simulink model "SAD_project"  (R2023b)
settings: Solver=ode4  StartTime=t0  StopTime=tf  FixedStep=t_step  RelTol=1e-3
model workspace (MAT data in the model file):
  N_order = 1
values from neighbouring files (symbols this model uses):
  A1 = importdata("igrfSg.txt")    [SAD_project_code.m]
  A2 = importdata("igrfSh.txt")    [SAD_project_code.m]
  A_1 = area_face(1)    [SAD_project_code.m]
  A_2 = area_face(2)    [SAD_project_code.m]
  A_3 = area_face(3)    [SAD_project_code.m]
  A_4 = area_face(4)    [SAD_project_code.m]
  A_5 = area_face(5)    [SAD_project_code.m]
  A_6 = area_face(6)    [SAD_project_code.m]
  alpha = [1/6 5/6]    [SAD_project_code.m]
  ARW = ARW*[1 1 1]'    [SAD_project_code.m]
  bias = bias*[1 1 1]'    [SAD_project_code.m]
  DCM_eci_per = rotationMatrix(rad2deg(i),rad2deg(OM), rad2deg(om))    [SAD_project_code.m]
  e = 0.0011241    [SAD_project_code.m]
  FS = 50000e-9    (= 5e-05)    [SAD_project_code.m]
  H0 = [g_10 g_11 h_11]'    [SAD_project_code.m]
  h_r_0 = [0,0,0]'    [SAD_project_code.m]
  horizon_cone_limit = deg2rad(350)    [SAD_project_code.m]
  i = deg2rad(97.55)    [SAD_project_code.m]
  I = 5/12.*diag([Ix Iy Iz])    [SAD_project_code.m]
  I_inv = inv(I)    [SAD_project_code.m]
  I_RW = 1e-2    (= 0.01)    [SAD_project_code.m]
  I_vector_RW = [I_RW I_RW I_RW]'    [SAD_project_code.m]
  inc_tot = sqrt(inc_lin^2 + inc_acc^2)    [SAD_project_code.m]
  InitialTrueAnomalyOfEarth = 0    [SAD_project_code.m]
  j_b = [0.001 0.005 0.001]'    [SAD_project_code.m]
  matrix_RW_config = eye(3)    [SAD_project_code.m]
  matrix_RW_config_inv = inv(matrix_RW_config)    [SAD_project_code.m]
  mu_E = astroConstants(13)    [SAD_project_code.m]
  N_1 = BODY(1,:)    [SAD_project_code.m]
  N_2 = BODY(2,:)    [SAD_project_code.m]
  N_3 = BODY(3,:)    [SAD_project_code.m]
  N_4 = BODY(4,:)    [SAD_project_code.m]
  N_5 = BODY(5,:)    [SAD_project_code.m]
  N_6 = BODY(6,:)    [SAD_project_code.m]
  n_e = sqrt(mu_E/a^3)    [SAD_project_code.m]
  om = deg2rad(206.3209)    [SAD_project_code.m]
  OM = deg2rad(50.7464)    [SAD_project_code.m]
  p = a*(1-e^2)    [SAD_project_code.m]
  q0 = [0.1, -0.7, 0.51, 0.41]    [SAD_project_code.m]
  r_1 = r(1,:)    [SAD_project_code.m]
  r_2 = r(2,:)    [SAD_project_code.m]
  r_3 = r(3,:)    [SAD_project_code.m]
  r_4 = r(4,:)    [SAD_project_code.m]
  r_5 = r(5,:)    [SAD_project_code.m]
  r_6 = r(6,:)    [SAD_project_code.m]
  R_E = astroConstants(23)    [SAD_project_code.m]
  rho_d1 = 0.1    [SAD_project_code.m]
  rho_d2 = 0.1    [SAD_project_code.m]
  rho_d3 = 0.1    [SAD_project_code.m]
  rho_d4 = 0.1    [SAD_project_code.m]
  rho_d5 = 0.1    [SAD_project_code.m]
  rho_d6 = 0.1    [SAD_project_code.m]
  rho_s1 = rho_s(1)    [SAD_project_code.m]
  rho_s2 = rho_s(2)    [SAD_project_code.m]
  rho_s3 = rho_s(3)    [SAD_project_code.m]
  rho_s4 = rho_s(4)    [SAD_project_code.m]
  rho_s5 = rho_s(5)    [SAD_project_code.m]
  rho_s6 = rho_s(6)    [SAD_project_code.m]
  t_step = 0.01    [SAD_project_code.m]
  th0 = deg2rad(0)    [SAD_project_code.m]
  timeoflaunch = date2mjd2000(date0)    [SAD_project_code.m]
  ts_sensor = 5*t_step    (= 0.05)    [SAD_project_code.m]
  w0 = [wx0 wy0 wz0]'    [SAD_project_code.m]
  w0_RW = [0 0 0]    [SAD_project_code.m]
  w_E = deg2rad(15.04)/60/60    [SAD_project_code.m]
  wMax_RW = 2*pi * RPM_max_RW / 60    (= 527.263967027)    [SAD_project_code.m]
libraries: matrix_library x21, simulink x5, simulink_extras x4, dspindex x3, vrlib x2, aerolibutil x1
(part 2 of 3)

== system SAD_project/Statistical methods attitude determination (quaternion  Wabha’s problem) /Vector z ==
  B : Inport
  Gain1 : Gain  Gain=-1
  Selector : Selector  NumberOfDimensions=2  InputPortWidth=3  IndexOptions=Index vector (dialog),Starting index (dialog)  Indices=2,3  OutputSizes=1,1
  Selector1 : Selector  NumberOfDimensions=2  InputPortWidth=3  IndexOptions=Index vector (dialog),Starting index (dialog)  Indices=1,3  OutputSizes=1,1
  Selector2 : Selector  NumberOfDimensions=2  InputPortWidth=3  IndexOptions=Index vector (dialog),Starting index (dialog)  Indices=1,2  OutputSizes=1,1
  Subtract1 : Sum  Inputs=+-
  Transpose1 : Math  Operator=transpose
  Vector Concatenate : Concatenate  NumInputs=3
  z : Outport
  wires:
  B/1 -> Subtract1/1, Transpose1/1
  Transpose1/1 -> Subtract1/2
  Selector2/1 -> Vector Concatenate/3
  Selector/1 -> Vector Concatenate/1
  Subtract1/1 -> Selector/1, Selector2/1, Selector1/1
  Vector Concatenate/1 -> z/1
  Gain1/1 -> Vector Concatenate/2
  Selector1/1 -> Gain1/1

== system SAD_project/Subsystem/Switch Case Action Adavanced Magnetic model ==
  r_N : Inport
  Action Port : ActionPort  PropagateVarSize=During execution  ActionPortLabel=case [ 1 ]:
  Advanced magnetic field model : Subsystem
  Constant : Constant  Value=N_order
  Gain : Gain  Gain=10^(-9)
  B_n : Outport  VectorParamsAs1DForOutWhenUnconnected=off
  wires:
  r_N/1 -> Advanced magnetic field model/1(r_N)
  Advanced magnetic field model/1(B_n) -> Gain/1
  Gain/1 -> B_n/1
  Constant/1 -> Advanced magnetic field model/2(N order)

== system SAD_project/Subsystem/Switch Case Action Dipole model ==
  r_N : Inport
  Action Port : ActionPort  PropagateVarSize=During execution  ActionPortLabel=default:
  Dipol Model of Magnetic Field : Subsystem
  Gain : Gain  Gain=10^(-9)
  "[g0_1, g1_1, h1_1]" : Constant  Value=H0
  b_N : Outport  VectorParamsAs1DForOutWhenUnconnected=off
  wires:
  "[g0_1, g1_1, h1_1]"/1 -> Dipol Model of Magnetic Field/1(H0 vector)
  r_N/1 -> Dipol Model of Magnetic Field/2(EarthSat_n)
  Dipol Model of Magnetic Field/1(b_N) -> Gain/1
  Gain/1 -> b_N/1

== system SAD_project/Sun sensor (Da fare sistmando vettore e eclissi)/Normalize Vector1 ==
  Vector : Inport
  Divide : Product  Inputs=*/
  Normalize Vector : Subsystem  AncestorBlock=LibrarySAD5/Normalize Vector1
  Versor : Outport
  wires:
  Vector/1 -> Normalize Vector/1(Vector), Divide/1
  Divide/1 -> Versor/1
  Normalize Vector/1(Norm) -> Divide/2

== system SAD_project/TRIAD: Attitude determination algebric Method with 2 sensor/Normalize Vector1 ==
  Vector : Inport
  Divide : Product  Inputs=*/
  Normalize Vector : Subsystem  AncestorBlock=LibrarySAD5/Normalize Vector1
  Versor : Outport
  wires:
  Vector/1 -> Normalize Vector/1(Vector), Divide/1
  Divide/1 -> Versor/1
  Normalize Vector/1(Norm) -> Divide/2

== system SAD_project/TRIAD: Attitude determination algebric Method with 2 sensor/Normalize Vector2 ==
  Vector : Inport
  Divide : Product  Inputs=*/
  Normalize Vector : Subsystem  AncestorBlock=LibrarySAD5/Normalize Vector1
  Versor : Outport
  wires:
  Vector/1 -> Normalize Vector/1(Vector), Divide/1
  Divide/1 -> Versor/1
  Normalize Vector/1(Norm) -> Divide/2

== system SAD_project/TRIAD: Attitude determination algebric Method with 2 sensor/Normalize Vector3 ==
  Vector : Inport
  Divide : Product  Inputs=*/
  Normalize Vector : Subsystem  AncestorBlock=LibrarySAD5/Normalize Vector1
  Versor : Outport
  wires:
  Vector/1 -> Normalize Vector/1(Vector), Divide/1
  Divide/1 -> Versor/1
  Normalize Vector/1(Norm) -> Divide/2

== system SAD_project/TRIAD: Attitude determination algebric Method with 2 sensor/Normalize Vector4 ==
  Vector : Inport
  Divide : Product  Inputs=*/
  Normalize Vector : Subsystem  AncestorBlock=LibrarySAD5/Normalize Vector1
  Versor : Outport
  wires:
  Vector/1 -> Normalize Vector/1(Vector), Divide/1
  Divide/1 -> Versor/1
  Normalize Vector/1(Norm) -> Divide/2

== system SAD_project/TRIAD: Attitude determination algebric Method with 2 sensor/Subsystem ==
  note: S1 = 𝑝;
      | 𝑠2 = (𝑝 ∧ 𝑞)/(|𝑝 ∧ 𝑞|);
      | 𝑠3 = 𝑝 ∧ 𝑠2
  versor p (body frame) : Inport
  versor q (body frame) : Inport  Port=2
  Cross Product : matrix_library/Cross Product
  Cross Product1 : matrix_library/Cross Product
  Matrix Concatenate : Concatenate  NumInputs=3  Mode=Multidimensional array  ConcatenateDimension=2
  Normalize Vector3 : Subsystem
  "Matrix S Measurements " : Outport
  wires:
  versor q (body frame)/1 -> Cross Product/2
  Normalize Vector3/1(Versor) -> Matrix Concatenate/2, Cross Product1/2  "s2"
  versor p (body frame)/1 -> Cross Product1/1, Matrix Concatenate/1, Cross Product/1  "s1"
  Cross Product/1 -> Normalize Vector3/1(Vector)
  Cross Product1/1 -> Matrix Concatenate/3  "s3"
  Matrix Concatenate/1 -> "Matrix S Measurements "/1  "Matrix of measure in body frame"

== system SAD_project/TRIAD: Attitude determination algebric Method with 2 sensor/Subsystem1 ==
  versor a (body frame) : Inport
  versor b (body frame) : Inport  Port=2
  Cross Product : matrix_library/Cross Product
  Cross Product1 : matrix_library/Cross Product
  Matrix Concatenate : Concatenate  NumInputs=3  Mode=Multidimensional array  ConcatenateDimension=2
  Normalize Vector3 : Subsystem
  "Matrix V certain model " : Outport
  wires:
  versor b (body frame)/1 -> Cross Product/2
  Normalize Vector3/1(Versor) -> Matrix Concatenate/2, Cross Product1/2  "s2"
  versor a (body frame)/1 -> Cross Product1/1, Matrix Concatenate/1, Cross Product/1  "s1"
  Cross Product/1 -> Normalize Vector3/1(Vector)
  Cross Product1/1 -> Matrix Concatenate/3  "s3"
  Matrix Concatenate/1 -> "Matrix V certain model "/1  "Matrix of measure in body frame"

== system SAD_project/two-body Keplerian dynamics ECI/Integretion of true anomaly ==
  th0 : Inport
  (1-e^2)^(3/2) : Subsystem
  Constant : Constant
  Cos : Trigonometry  Operator=cos
  Divide : Product  Inputs=*/
  Gain : Gain  Gain=e
  Gain1 : Gain  Gain=n_e
  Integrator : Integrator  InitialConditionSource=external
  Product : Product
  Sum : Sum  Inputs=|++
  th : Outport
  wires:
  Sum/1 -> Product/1, Product/2
  Integrator/1 -> th/1, Cos/1  "theta"
  Divide/1 -> Integrator/1
  Constant/1 -> Sum/1
  Product/1 -> Gain1/1
  Cos/1 -> Gain/1
  Gain/1 -> Sum/2
  (1-e^2)^(3/2)/1(Out1) -> Divide/2
  th0/1 -> Integrator/2
  Gain1/1 -> Divide/1

== system SAD_project/two-body Keplerian dynamics ECI/r_perifocal ==
  th : Inport
  Calculation of norm r : Subsystem
  Constant : Constant  Value=0
  Cos : Trigonometry  Operator=cos
  Mux : Mux  Inputs=3
  Product : Product
  Sin : Trigonometry
  r_per : Outport
  wires:
  Constant/1 -> Mux/3
  Cos/1 -> Mux/1
  th/1 -> Calculation of norm r/1(th), Cos/1, Sin/1
  Sin/1 -> Mux/2
  Mux/1 -> Product/1  "r_n"
  Calculation of norm r/1(Norm(r)) -> Product/2
  Product/1 -> r_per/1  "r_n"

== system SAD_project/Calculation of disturbance torque/M of gravity gradient1/Norm of vector ==
  Vector : Inport
  Dot Product : DotProduct  OutDataTypeStr=Inherit: Inherit via internal rule
  Sqrt : Sqrt
  Norm : Outport
  wires:
  Sqrt/1 -> Norm/1
  Vector/1 -> Dot Product/1, Dot Product/2
  Dot Product/1 -> Sqrt/1

== system SAD_project/Calculation of disturbance torque/Solar pressure on 6 faces/Norm of vector ==
  Vector : Inport
  Dot Product : DotProduct  OutDataTypeStr=Inherit: Inherit via internal rule
  Sqrt : Sqrt
  Norm : Outport
  wires:
  Sqrt/1 -> Norm/1
  Vector/1 -> Dot Product/1, Dot Product/2
  Dot Product/1 -> Sqrt/1

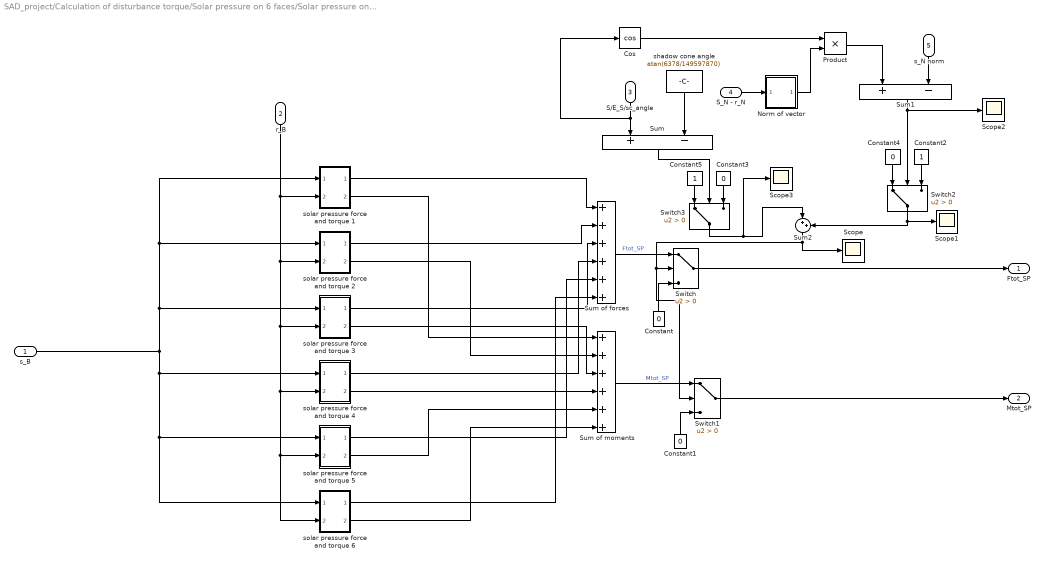
== system SAD_project/Calculation of disturbance torque/Solar pressure on 6 faces/Solar pressure on 6 faces1 ==
  s_B : Inport
  r_B : Inport  Port=2
  S/E_S/sc_angle : Inport  Port=3
  S_N - r_N : Inport  Port=4
  s_N norm : Inport  Port=5
  Constant{,1,3..4} (4 alike) : Constant  Value=0
  Constant2 : Constant
  Constant5 : Constant
  Cos : Trigonometry  Operator=cos
  Norm of vector : Subsystem  AncestorBlock=LibrarySAD5/Normalize Vector1
  Product : Product
  Scope{,1..3} (4 alike) : Scope
  Sum : Sum  Inputs=+-
  Sum of forces : Sum  Inputs=++++++
  Sum of moments : Sum  Inputs=++++++
  Sum1 : Sum  Inputs=+-
  Sum2 : Sum  Inputs=|++
  Switch{,1..3} (4 alike) : Switch  Criteria=u2 > Threshold  SaturateOnIntegerOverflow=off  InputSameDT=off
  shadow cone angle : Constant  Value=atan(6378/149597870)
  solar pressure force and torque 1 : Subsystem
  solar pressure force and torque 2 : Subsystem
  solar pressure force and torque 3 : Subsystem
  solar pressure force and torque 4 : Subsystem
  solar pressure force and torque 5 : Subsystem
  solar pressure force and torque 6 : Subsystem
  Ftot_SP : Outport
  Mtot_SP : Outport  Port=2
  wires:
  s_B/1 -> solar pressure force and torque 1/1(s_B), solar pressure force and torque 2/1(s_B), solar pressure force and torque 3/1(s_B), solar pressure force and torque 4/1(s_B), solar pressure force and torque 6/1(s_B), solar pressure force and torque 5/1(s_B)
  solar pressure force and torque 1/1(F_1) -> Sum of forces/1
  solar pressure force and torque 1/2(M_1) -> Sum of moments/1
  solar pressure force and torque 2/1(F_2) -> Sum of forces/2
  r_B/1 -> solar pressure force and torque 6/2(r_N), solar pressure force and torque 5/2(r_N), solar pressure force and torque 4/2(r_N), solar pressure force and torque 3/2(r_N), solar pressure force and torque 2/2(r_N), solar pressure force and torque 1/2(r_N)
  solar pressure force and torque 2/2(M_2) -> Sum of moments/2
  solar pressure force and torque 3/1(F_3) -> Sum of forces/3
  solar pressure force and torque 3/2(M_3) -> Sum of moments/3
  solar pressure force and torque 4/1(F_4) -> Sum of forces/4
  solar pressure force and torque 4/2(M_4) -> Sum of moments/4
  solar pressure force and torque 5/1(F_5) -> Sum of forces/5
  solar pressure force and torque 5/2(M_5) -> Sum of moments/5
  solar pressure force and torque 6/1(F_6) -> Sum of forces/6
  solar pressure force and torque 6/2(M_6) -> Sum of moments/6
  Sum of forces/1 -> Switch/1  "Ftot_SP"
  Constant/1 -> Switch/3
  S/E_S/sc_angle/1 -> Cos/1, Sum/1
  shadow cone angle/1 -> Sum/2
  Sum of moments/1 -> Switch1/1  "Mtot_SP"
  Constant1/1 -> Switch1/3
  S_N - r_N/1 -> Norm of vector/1(Vector)
  Constant2/1 -> Switch2/3
  Cos/1 -> Product/1
  Norm of vector/1(Norm) -> Product/2
  Product/1 -> Sum1/1
  s_N norm/1 -> Sum1/2
  Sum/1 -> Switch3/2
  Sum1/1 -> Switch2/2, Scope2/1
  Constant4/1 -> Switch2/1
  Constant5/1 -> Switch3/1
  Constant3/1 -> Switch3/3
  Switch3/1 -> Scope3/1, Sum2/1
  Switch2/1 -> Sum2/2, Scope1/1
  Sum2/1 -> Scope/1, Switch1/2, Switch/2
  Switch/1 -> Ftot_SP/1
  Switch1/1 -> Mtot_SP/1

== system SAD_project/Create matrix to statistical method/Normalize Vector1/Normalize Vector ==
  Vector : Inport
  Dot Product : DotProduct  OutDataTypeStr=Inherit: Inherit via internal rule
  Sqrt : Sqrt
  Norm : Outport
  wires:
  Sqrt/1 -> Norm/1
  Vector/1 -> Dot Product/1, Dot Product/2
  Dot Product/1 -> Sqrt/1

== system SAD_project/Create matrix to statistical method/Normalize Vector2/Normalize Vector ==
  Vector : Inport
  Dot Product : DotProduct  OutDataTypeStr=Inherit: Inherit via internal rule
  Sqrt : Sqrt
  Norm : Outport
  wires:
  Sqrt/1 -> Norm/1
  Vector/1 -> Dot Product/1, Dot Product/2
  Dot Product/1 -> Sqrt/1

== system SAD_project/Create matrix to statistical method/Normalize Vector3/Normalize Vector ==
  Vector : Inport
  Dot Product : DotProduct  OutDataTypeStr=Inherit: Inherit via internal rule
  Sqrt : Sqrt
  Norm : Outport
  wires:
  Sqrt/1 -> Norm/1
  Vector/1 -> Dot Product/1, Dot Product/2
  Dot Product/1 -> Sqrt/1

== system SAD_project/Create matrix to statistical method/Normalize Vector4/Normalize Vector ==
  Vector : Inport
  Dot Product : DotProduct  OutDataTypeStr=Inherit: Inherit via internal rule
  Sqrt : Sqrt
  Norm : Outport
  wires:
  Sqrt/1 -> Norm/1
  Vector/1 -> Dot Product/1, Dot Product/2
  Dot Product/1 -> Sqrt/1

== system SAD_project/Dynamics e Kinematics/Attitude error GG/calculating A_B//L ==
  Theta : Inport
  A_B/N : Inport  Port=2
  Matrix Multiply : Product  Multiplication=Matrix(*)
  Subsystem : Subsystem
  Transpose : Math  Operator=transpose
  A_B/L : Outport
  wires:
  Theta/1 -> Subsystem/1(Theta)
  Transpose/1 -> Matrix Multiply/2
  A_B/N/1 -> Matrix Multiply/1
  Matrix Multiply/1 -> A_B/L/1
  Subsystem/1(" A_L/N") -> Transpose/1

== system SAD_project/Dynamics e Kinematics/DCM composition from quaternions 1/Cross product matrix composition ==
  q_vect : Inport
  Demux : Demux  Outputs=3
  Gain : Gain  Gain=[0 0 0; 0 0 -1; 0 1 0]
  Gain1 : Gain  Gain=[0 0 1; 0 0 0; -1 0 0]
  Gain2 : Gain  Gain=[0 -1 0; 1 0 0; 0 0 0]
  Sum : Sum  Inputs=+++
  q_vect cross : Outport
  wires:
  Gain1/1 -> Sum/2
  Demux/3 -> Gain2/1
  Demux/1 -> Gain/1
  q_vect/1 -> Demux/1
  Gain2/1 -> Sum/3
  Demux/2 -> Gain1/1
  Gain/1 -> Sum/1
  Sum/1 -> q_vect cross/1

== system SAD_project/Dynamics e Kinematics/Kinematics quaternion2/Matrix OMEGA ==
  omega : Inport
  Constant4 : Constant  Value=0
  Demux : Demux  Outputs=3
  Gain : Gain  Gain=-1
  Gain1 : Gain  Gain=-1
  Gain2 : Gain  Gain=-1
  Matrix Concatenate : Concatenate  NumInputs=4  Mode=Multidimensional array  ConcatenateDimension=2
  Vector Concatenate{,2..4} (4 alike) : Concatenate  NumInputs=4
  Matrix Omega : Outport
  wires:
  Demux/2 -> Vector Concatenate4/2, Vector Concatenate/3, Gain1/1  "W_v"
  Gain1/1 -> Vector Concatenate2/4, Vector Concatenate3/1
  Matrix Concatenate/1 -> Matrix Omega/1
  Gain2/1 -> Vector Concatenate3/4, Vector Concatenate/2  "-W_w"
  Vector Concatenate3/1 -> Matrix Concatenate/3
  Demux/3 -> Vector Concatenate2/1, Vector Concatenate4/3, Gain2/1  "W_w"
  Gain/1 -> Vector Concatenate/4, Vector Concatenate2/3  "-W_u"
  Constant4/1 -> Vector Concatenate/1, Vector Concatenate2/2, Vector Concatenate3/3, Vector Concatenate4/4
  Demux/1 -> Vector Concatenate3/2, Vector Concatenate4/1, Gain/1  "W_u"
  Vector Concatenate4/1 -> Matrix Concatenate/4
  Vector Concatenate2/1 -> Matrix Concatenate/2
  Vector Concatenate/1 -> Matrix Concatenate/1
  omega/1 -> Demux/1

== system SAD_project/Dynamics e Kinematics/Kinematics quaternion2/Normalize Vector2 ==
  Vector : Inport
  Dot Product : DotProduct  OutDataTypeStr=Inherit: Inherit via internal rule
  Sqrt : Sqrt
  Norm : Outport
  wires:
  Sqrt/1 -> Norm/1
  Vector/1 -> Dot Product/1, Dot Product/2
  Dot Product/1 -> Sqrt/1

== system SAD_project/Horizon Sensor/Normalize Vector1/Normalize Vector ==
  Vector : Inport
  Dot Product : DotProduct  OutDataTypeStr=Inherit: Inherit via internal rule
  Sqrt : Sqrt
  Norm : Outport
  wires:
  Sqrt/1 -> Norm/1
  Vector/1 -> Dot Product/1, Dot Product/2
  Dot Product/1 -> Sqrt/1

== system SAD_project/Subsystem/Switch Case Action Adavanced Magnetic model/Advanced magnetic field model ==
  note: INPUT:
      | - r_N are the coordinates of the satellite in the ECI frame
      | - A_bn is the DCM matrix to change from inertial frame to body frame
      | - timeoflaunch is the julian time at the start of simulation
      | - A1 and A2 are the matrices containing the coefficients of g and h up to the 13th order
      | - j_B is the residual magnetic induction
  note: the timeoflaunch is corrected by adding the time of simulation using a clock
  r_N : Inport
  N order : Inport  Port=2
  Clock1 : Clock
  Constant21 : Constant  Value=timeoflaunch
  Constant23 : Constant  Value=A1
  Constant24 : Constant  Value=A2
  Gain1 : Gain  Gain=1/(3600*24)
  MATLAB Function : MATLAB Function  TreatAsAtomicUnit=on
  Product3 : Product  Multiplication=Matrix(*)
  Rotation matrix for earth spin : Subsystem
  Sum : Sum  Inputs=|++
  cart to sph coord : Subsystem
  B_n : Outport
  wires:
  Rotation matrix for earth spin/1(eci_to_ecef) -> Product3/1
  Clock1/1 -> Gain1/1
  r_N/1 -> Product3/2
  Constant24/1 -> MATLAB Function/7(A2)
  cart to sph coord/3(long) -> MATLAB Function/4(LST), MATLAB Function/3(phi)
  Constant23/1 -> MATLAB Function/6(A1)
  Gain1/1 -> Sum/2
  Product3/1 -> cart to sph coord/1(r_xyz)
  cart to sph coord/2(lat) -> MATLAB Function/2(theta)
  Constant21/1 -> Sum/1
  Sum/1 -> MATLAB Function/5(mjd2000)
  cart to sph coord/1(r) -> MATLAB Function/1(r)
  MATLAB Function/1(B_n) -> B_n/1
  N order/1 -> MATLAB Function/8(N)

== system SAD_project/Subsystem/Switch Case Action Dipole model/Dipol Model of Magnetic Field ==
  note: CODE TO ADD
      | % Definition of Magnetic Field (Dipole model)
      |  j_b = [0.01 0.05 0.01]';
      | H0 = 1e-9.*[-29404.8 -1450.9 4652.5]';
  H0 vector : Inport
  EarthSat_n : Inport  Port=2
  Calculation of b_n : Subsystem
  b_N : Outport
  wires:
  H0 vector/1 -> Calculation of b_n/1(H0 vector)
  EarthSat_n/1 -> Calculation of b_n/2(EarthSat_n)
  Calculation of b_n/1(b_N) -> b_N/1

== system SAD_project/Sun sensor (Da fare sistmando vettore e eclissi)/Normalize Vector1/Normalize Vector ==
  Vector : Inport
  Dot Product : DotProduct  OutDataTypeStr=Inherit: Inherit via internal rule
  Sqrt : Sqrt
  Norm : Outport
  wires:
  Sqrt/1 -> Norm/1
  Vector/1 -> Dot Product/1, Dot Product/2
  Dot Product/1 -> Sqrt/1

== system SAD_project/TRIAD: Attitude determination algebric Method with 2 sensor/Normalize Vector1/Normalize Vector ==
  Vector : Inport
  Dot Product : DotProduct  OutDataTypeStr=Inherit: Inherit via internal rule
  Sqrt : Sqrt
  Norm : Outport
  wires:
  Sqrt/1 -> Norm/1
  Vector/1 -> Dot Product/1, Dot Product/2
  Dot Product/1 -> Sqrt/1

== system SAD_project/TRIAD: Attitude determination algebric Method with 2 sensor/Normalize Vector2/Normalize Vector ==
  Vector : Inport
  Dot Product : DotProduct  OutDataTypeStr=Inherit: Inherit via internal rule
  Sqrt : Sqrt
  Norm : Outport
  wires:
  Sqrt/1 -> Norm/1
  Vector/1 -> Dot Product/1, Dot Product/2
  Dot Product/1 -> Sqrt/1

== system SAD_project/TRIAD: Attitude determination algebric Method with 2 sensor/Normalize Vector3/Normalize Vector ==
  Vector : Inport
  Dot Product : DotProduct  OutDataTypeStr=Inherit: Inherit via internal rule
  Sqrt : Sqrt
  Norm : Outport
  wires:
  Sqrt/1 -> Norm/1
  Vector/1 -> Dot Product/1, Dot Product/2
  Dot Product/1 -> Sqrt/1

== system SAD_project/TRIAD: Attitude determination algebric Method with 2 sensor/Normalize Vector4/Normalize Vector ==
  Vector : Inport
  Dot Product : DotProduct  OutDataTypeStr=Inherit: Inherit via internal rule
  Sqrt : Sqrt
  Norm : Outport
  wires:
  Sqrt/1 -> Norm/1
  Vector/1 -> Dot Product/1, Dot Product/2
  Dot Product/1 -> Sqrt/1

== system SAD_project/TRIAD: Attitude determination algebric Method with 2 sensor/Subsystem/Normalize Vector3 ==
  Vector : Inport
  Divide : Product  Inputs=*/
  Normalize Vector : Subsystem  AncestorBlock=LibrarySAD5/Normalize Vector1
  Versor : Outport
  wires:
  Vector/1 -> Normalize Vector/1(Vector), Divide/1
  Divide/1 -> Versor/1
  Normalize Vector/1(Norm) -> Divide/2

== system SAD_project/TRIAD: Attitude determination algebric Method with 2 sensor/Subsystem1/Normalize Vector3 ==
  Vector : Inport
  Divide : Product  Inputs=*/
  Normalize Vector : Subsystem  AncestorBlock=LibrarySAD5/Normalize Vector1
  Versor : Outport
  wires:
  Vector/1 -> Normalize Vector/1(Vector), Divide/1
  Divide/1 -> Versor/1
  Normalize Vector/1(Norm) -> Divide/2

== system SAD_project/two-body Keplerian dynamics ECI/Integretion of true anomaly/(1-e^2)^(3//2) ==
  Constant1 : Constant
  Constant2 : Constant  Value=e
  Constant3 : Constant  Value=3/2
  Power : Math  Operator=pow
  Product1 : Product
  Subtract : Sum  Inputs=+-
  Out1 : Outport
  wires:
  Constant3/1 -> Power/2
  Constant2/1 -> Product1/2, Product1/1
  Subtract/1 -> Power/1
  Constant1/1 -> Subtract/1
  Product1/1 -> Subtract/2
  Power/1 -> Out1/1

== system SAD_project/two-body Keplerian dynamics ECI/r_perifocal/Calculation of norm r ==
  th : Inport
  Constant : Constant  Value=p
  Constant2 : Constant
  Cos : Trigonometry  Operator=cos
  Divide : Product  Inputs=*/
  Gain1 : Gain  Gain=e
  Sum : Sum  Inputs=|++
  Norm(r) : Outport
  wires:
  Constant/1 -> Divide/1
  Gain1/1 -> Sum/2
  Constant2/1 -> Sum/1
  Cos/1 -> Gain1/1
  Sum/1 -> Divide/2
  th/1 -> Cos/1
  Divide/1 -> Norm(r)/1

== system SAD_project/Calculation of disturbance torque/Solar pressure on 6 faces/Solar pressure on 6 faces1/Norm of vector ==
  Vector : Inport
  Dot Product : DotProduct  OutDataTypeStr=Inherit: Inherit via internal rule
  Sqrt : Sqrt
  Norm : Outport
  wires:
  Sqrt/1 -> Norm/1
  Vector/1 -> Dot Product/1, Dot Product/2
  Dot Product/1 -> Sqrt/1

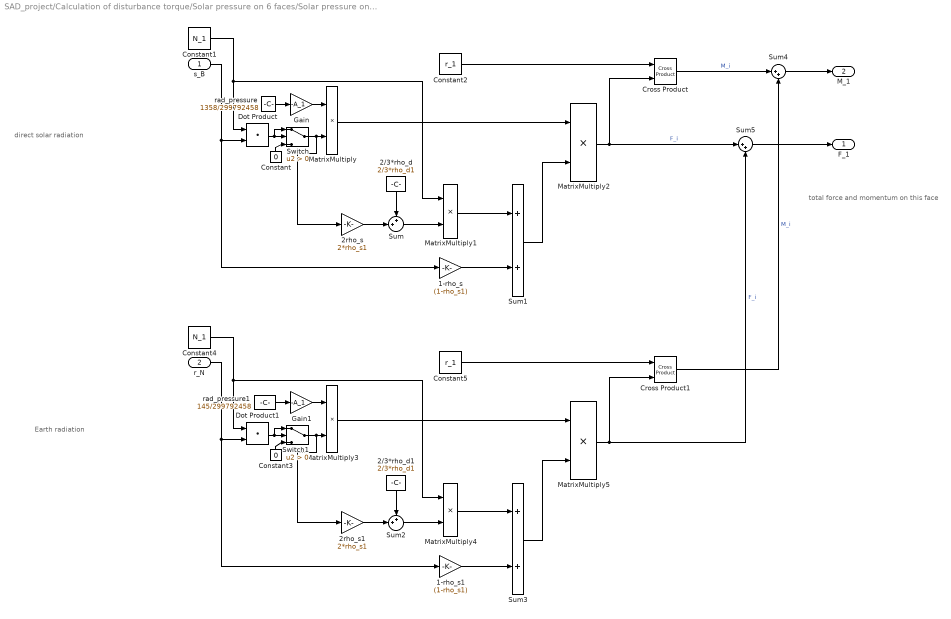
== system SAD_project/Calculation of disturbance torque/Solar pressure on 6 faces/Solar pressure on 6 faces1/solar pressure force and torque 1 ==
  note: total force and
      | momentum on this face
  note: direct solar radiation
  note: Earth radiation
  s_B : Inport
  r_N : Inport  Port=2
  1-rho_s : Gain  Gain=(1-rho_s1)
  1-rho_s1 : Gain  Gain=(1-rho_s1)
  2/3*rho_d : Constant  Value=2/3*rho_d1
  2/3*rho_d1 : Constant  Value=2/3*rho_d1
  2rho_s : Gain  Gain=2*rho_s1
  2rho_s1 : Gain  Gain=2*rho_s1
  Constant : Constant  Value=0
  Constant1 : Constant  Value=N_1
  Constant2 : Constant  Value=r_1
  Constant3 : Constant  Value=0
  Constant4 : Constant  Value=N_1
  Constant5 : Constant  Value=r_1
  Cross Product : matrix_library/Cross Product
  Cross Product1 : matrix_library/Cross Product
  Dot Product : DotProduct  OutDataTypeStr=Inherit: Inherit via internal rule
  Dot Product1 : DotProduct  OutDataTypeStr=Inherit: Inherit via internal rule
  Gain : Gain  Gain=-A_1
  Gain1 : Gain  Gain=-A_1
  MatrixMultiply{,1..5} (6 alike) : Product
  Sum : Sum  Inputs=++|
  Sum1 : Sum
  Sum2 : Sum  Inputs=++|
  Sum3 : Sum
  Sum4 : Sum  Inputs=|++
  Sum5 : Sum  Inputs=|++
  Switch : Switch  Criteria=u2 > Threshold  SaturateOnIntegerOverflow=off  InputSameDT=off
  Switch1 : Switch  Criteria=u2 > Threshold  SaturateOnIntegerOverflow=off  InputSameDT=off
  rad_pressure : Constant  Value=1358/299792458
  rad_pressure1 : Constant  Value=145/299792458
  F_1 : Outport
  M_1 : Outport  Port=2
  wires:
  MatrixMultiply2/1 -> Sum5/1, Cross Product/2  "F_i"
  MatrixMultiply/1 -> MatrixMultiply2/1
  Sum1/1 -> MatrixMultiply2/2
  s_B/1 -> 1-rho_s/1, Dot Product/2
  1-rho_s/1 -> Sum1/2
  rad_pressure/1 -> Gain/1
  MatrixMultiply1/1 -> Sum1/1
  Constant1/1 -> MatrixMultiply1/1, Dot Product/1
  Gain/1 -> MatrixMultiply/1
  Constant2/1 -> Cross Product/1
  Dot Product/1 -> Switch/1, Switch/2
  Constant/1 -> Switch/3
  Switch/1 -> 2rho_s/1, MatrixMultiply/2
  2rho_s/1 -> Sum/2
  2/3*rho_d/1 -> Sum/1
  Sum/1 -> MatrixMultiply1/2
  Sum3/1 -> MatrixMultiply5/2
  r_N/1 -> 1-rho_s1/1, Dot Product1/2
  1-rho_s1/1 -> Sum3/2
  2rho_s1/1 -> Sum2/2
  Switch1/1 -> 2rho_s1/1, MatrixMultiply3/2
  MatrixMultiply4/1 -> Sum3/1
  Constant5/1 -> Cross Product1/1
  MatrixMultiply3/1 -> MatrixMultiply5/1
  rad_pressure1/1 -> Gain1/1
  Constant3/1 -> Switch1/3
  Constant4/1 -> MatrixMultiply4/1, Dot Product1/1
  MatrixMultiply5/1 -> Sum5/2, Cross Product1/2  "F_i"
  Dot Product1/1 -> Switch1/1, Switch1/2
  Cross Product1/1 -> Sum4/2  "M_i"
  Sum2/1 -> MatrixMultiply4/2
  Gain1/1 -> MatrixMultiply3/1
  2/3*rho_d1/1 -> Sum2/1
  Sum4/1 -> M_1/1
  Cross Product/1 -> Sum4/1  "M_i"
  Sum5/1 -> F_1/1

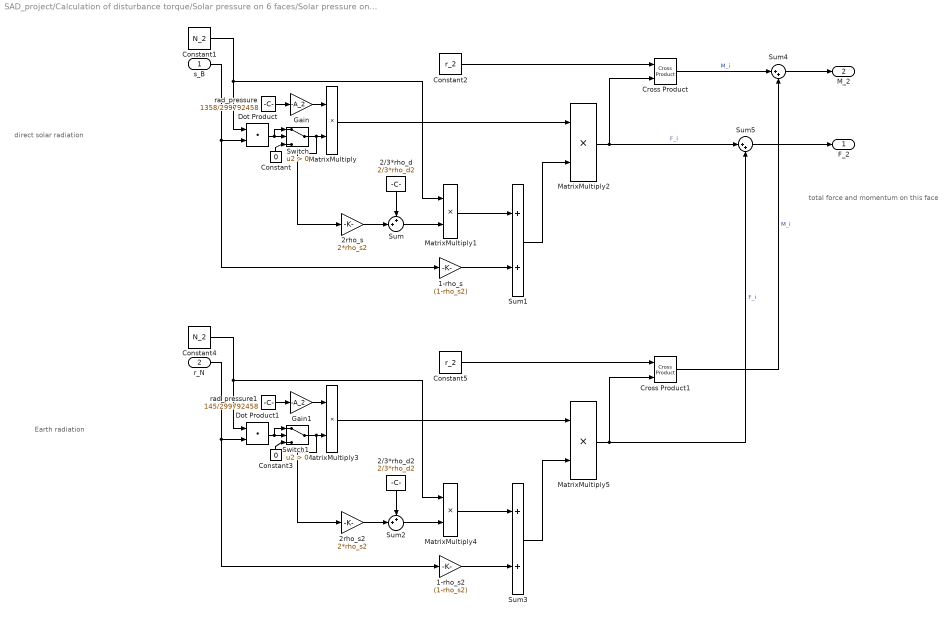
== system SAD_project/Calculation of disturbance torque/Solar pressure on 6 faces/Solar pressure on 6 faces1/solar pressure force and torque 2 ==
  note: total force and
      | momentum on this face
  note: direct solar radiation
  note: Earth radiation
  s_B : Inport
  r_N : Inport  Port=2
  1-rho_s : Gain  Gain=(1-rho_s2)
  1-rho_s2 : Gain  Gain=(1-rho_s2)
  2/3*rho_d : Constant  Value=2/3*rho_d2
  2/3*rho_d2 : Constant  Value=2/3*rho_d2
  2rho_s : Gain  Gain=2*rho_s2
  2rho_s2 : Gain  Gain=2*rho_s2
  Constant : Constant  Value=0
  Constant1 : Constant  Value=N_2
  Constant2 : Constant  Value=r_2
  Constant3 : Constant  Value=0
  Constant4 : Constant  Value=N_2
  Constant5 : Constant  Value=r_2
  Cross Product : matrix_library/Cross Product
  Cross Product1 : matrix_library/Cross Product
  Dot Product : DotProduct  OutDataTypeStr=Inherit: Inherit via internal rule
  Dot Product1 : DotProduct  OutDataTypeStr=Inherit: Inherit via internal rule
  Gain : Gain  Gain=-A_2
  Gain1 : Gain  Gain=-A_2
  MatrixMultiply{,1..5} (6 alike) : Product
  Sum : Sum  Inputs=++|
  Sum1 : Sum
  Sum2 : Sum  Inputs=++|
  Sum3 : Sum
  Sum4 : Sum  Inputs=|++
  Sum5 : Sum  Inputs=|++
  Switch : Switch  Criteria=u2 > Threshold  SaturateOnIntegerOverflow=off  InputSameDT=off
  Switch1 : Switch  Criteria=u2 > Threshold  SaturateOnIntegerOverflow=off  InputSameDT=off
  rad_pressure : Constant  Value=1358/299792458
  rad_pressure1 : Constant  Value=145/299792458
  F_2 : Outport
  M_2 : Outport  Port=2
  wires:
  MatrixMultiply2/1 -> Sum5/1, Cross Product/2  "F_i"
  MatrixMultiply/1 -> MatrixMultiply2/1
  Sum1/1 -> MatrixMultiply2/2
  s_B/1 -> 1-rho_s/1, Dot Product/2
  1-rho_s/1 -> Sum1/2
  rad_pressure/1 -> Gain/1
  MatrixMultiply1/1 -> Sum1/1
  Constant1/1 -> MatrixMultiply1/1, Dot Product/1
  Gain/1 -> MatrixMultiply/1
  Constant2/1 -> Cross Product/1
  Dot Product/1 -> Switch/1, Switch/2
  Constant/1 -> Switch/3
  Switch/1 -> 2rho_s/1, MatrixMultiply/2
  2rho_s/1 -> Sum/2
  2/3*rho_d/1 -> Sum/1
  Sum/1 -> MatrixMultiply1/2
  Sum3/1 -> MatrixMultiply5/2
  r_N/1 -> 1-rho_s2/1, Dot Product1/2
  1-rho_s2/1 -> Sum3/2
  2rho_s2/1 -> Sum2/2
  Switch1/1 -> 2rho_s2/1, MatrixMultiply3/2
  MatrixMultiply4/1 -> Sum3/1
  Constant5/1 -> Cross Product1/1
  MatrixMultiply3/1 -> MatrixMultiply5/1
  rad_pressure1/1 -> Gain1/1
  Constant3/1 -> Switch1/3
  Constant4/1 -> MatrixMultiply4/1, Dot Product1/1
  MatrixMultiply5/1 -> Sum5/2, Cross Product1/2  "F_i"
  Dot Product1/1 -> Switch1/1, Switch1/2
  Cross Product1/1 -> Sum4/2  "M_i"
  Sum2/1 -> MatrixMultiply4/2
  Gain1/1 -> MatrixMultiply3/1
  2/3*rho_d2/1 -> Sum2/1
  Sum4/1 -> M_2/1
  Cross Product/1 -> Sum4/1  "M_i"
  Sum5/1 -> F_2/1

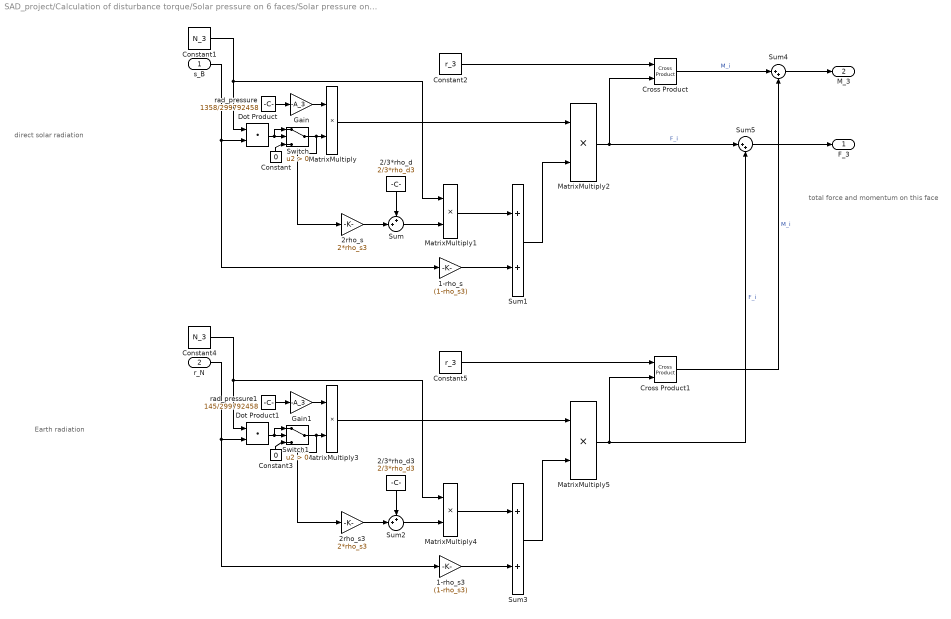
== system SAD_project/Calculation of disturbance torque/Solar pressure on 6 faces/Solar pressure on 6 faces1/solar pressure force and torque 3 ==
  note: total force and
      | momentum on this face
  note: direct solar radiation
  note: Earth radiation
  s_B : Inport
  r_N : Inport  Port=2
  1-rho_s : Gain  Gain=(1-rho_s3)
  1-rho_s3 : Gain  Gain=(1-rho_s3)
  2/3*rho_d : Constant  Value=2/3*rho_d3
  2/3*rho_d3 : Constant  Value=2/3*rho_d3
  2rho_s : Gain  Gain=2*rho_s3
  2rho_s3 : Gain  Gain=2*rho_s3
  Constant : Constant  Value=0
  Constant1 : Constant  Value=N_3
  Constant2 : Constant  Value=r_3
  Constant3 : Constant  Value=0
  Constant4 : Constant  Value=N_3
  Constant5 : Constant  Value=r_3
  Cross Product : matrix_library/Cross Product
  Cross Product1 : matrix_library/Cross Product
  Dot Product : DotProduct  OutDataTypeStr=Inherit: Inherit via internal rule
  Dot Product1 : DotProduct  OutDataTypeStr=Inherit: Inherit via internal rule
  Gain : Gain  Gain=-A_3
  Gain1 : Gain  Gain=-A_3
  MatrixMultiply{,1..5} (6 alike) : Product
  Sum : Sum  Inputs=++|
  Sum1 : Sum
  Sum2 : Sum  Inputs=++|
  Sum3 : Sum
  Sum4 : Sum  Inputs=|++
  Sum5 : Sum  Inputs=|++
  Switch : Switch  Criteria=u2 > Threshold  SaturateOnIntegerOverflow=off  InputSameDT=off
  Switch1 : Switch  Criteria=u2 > Threshold  SaturateOnIntegerOverflow=off  InputSameDT=off
  rad_pressure : Constant  Value=1358/299792458
  rad_pressure1 : Constant  Value=145/299792458
  F_3 : Outport
  M_3 : Outport  Port=2
  wires:
  MatrixMultiply2/1 -> Sum5/1, Cross Product/2  "F_i"
  MatrixMultiply/1 -> MatrixMultiply2/1
  Sum1/1 -> MatrixMultiply2/2
  s_B/1 -> 1-rho_s/1, Dot Product/2
  1-rho_s/1 -> Sum1/2
  rad_pressure/1 -> Gain/1
  MatrixMultiply1/1 -> Sum1/1
  Constant1/1 -> MatrixMultiply1/1, Dot Product/1
  Gain/1 -> MatrixMultiply/1
  Constant2/1 -> Cross Product/1
  Dot Product/1 -> Switch/1, Switch/2
  Constant/1 -> Switch/3
  Switch/1 -> 2rho_s/1, MatrixMultiply/2
  2rho_s/1 -> Sum/2
  2/3*rho_d/1 -> Sum/1
  Sum/1 -> MatrixMultiply1/2
  Sum3/1 -> MatrixMultiply5/2
  r_N/1 -> 1-rho_s3/1, Dot Product1/2
  1-rho_s3/1 -> Sum3/2
  2rho_s3/1 -> Sum2/2
  Switch1/1 -> 2rho_s3/1, MatrixMultiply3/2
  MatrixMultiply4/1 -> Sum3/1
  Constant5/1 -> Cross Product1/1
  MatrixMultiply3/1 -> MatrixMultiply5/1
  rad_pressure1/1 -> Gain1/1
  Constant3/1 -> Switch1/3
  Constant4/1 -> MatrixMultiply4/1, Dot Product1/1
  MatrixMultiply5/1 -> Sum5/2, Cross Product1/2  "F_i"
  Dot Product1/1 -> Switch1/1, Switch1/2
  Cross Product1/1 -> Sum4/2  "M_i"
  Sum2/1 -> MatrixMultiply4/2
  Gain1/1 -> MatrixMultiply3/1
  2/3*rho_d3/1 -> Sum2/1
  Sum4/1 -> M_3/1
  Cross Product/1 -> Sum4/1  "M_i"
  Sum5/1 -> F_3/1

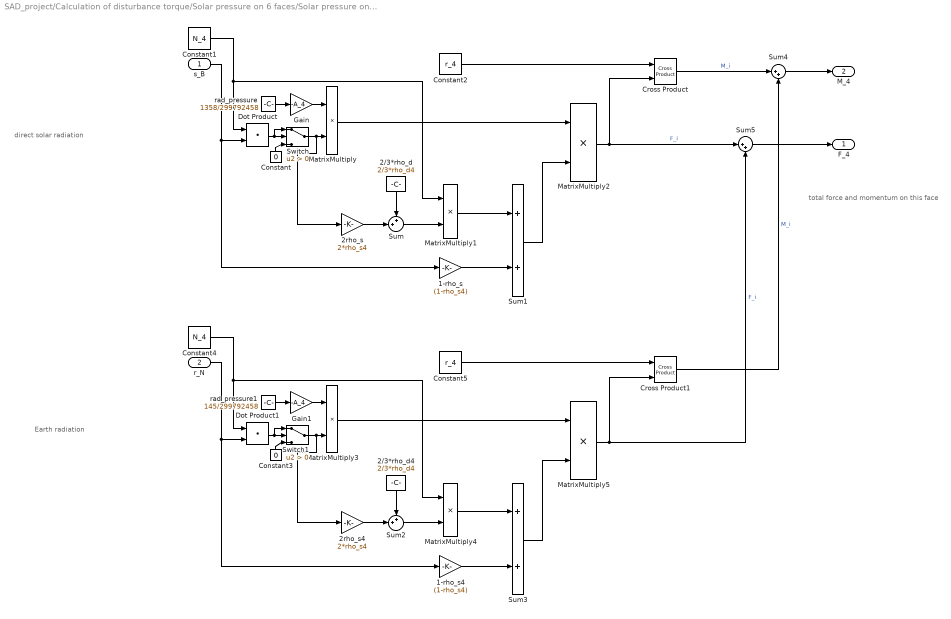
== system SAD_project/Calculation of disturbance torque/Solar pressure on 6 faces/Solar pressure on 6 faces1/solar pressure force and torque 4 ==
  note: total force and
      | momentum on this face
  note: direct solar radiation
  note: Earth radiation
  s_B : Inport
  r_N : Inport  Port=2
  1-rho_s : Gain  Gain=(1-rho_s4)
  1-rho_s4 : Gain  Gain=(1-rho_s4)
  2/3*rho_d : Constant  Value=2/3*rho_d4
  2/3*rho_d4 : Constant  Value=2/3*rho_d4
  2rho_s : Gain  Gain=2*rho_s4
  2rho_s4 : Gain  Gain=2*rho_s4
  Constant : Constant  Value=0
  Constant1 : Constant  Value=N_4
  Constant2 : Constant  Value=r_4
  Constant3 : Constant  Value=0
  Constant4 : Constant  Value=N_4
  Constant5 : Constant  Value=r_4
  Cross Product : matrix_library/Cross Product
  Cross Product1 : matrix_library/Cross Product
  Dot Product : DotProduct  OutDataTypeStr=Inherit: Inherit via internal rule
  Dot Product1 : DotProduct  OutDataTypeStr=Inherit: Inherit via internal rule
  Gain : Gain  Gain=-A_4
  Gain1 : Gain  Gain=-A_4
  MatrixMultiply{,1..5} (6 alike) : Product
  Sum : Sum  Inputs=++|
  Sum1 : Sum
  Sum2 : Sum  Inputs=++|
  Sum3 : Sum
  Sum4 : Sum  Inputs=|++
  Sum5 : Sum  Inputs=|++
  Switch : Switch  Criteria=u2 > Threshold  SaturateOnIntegerOverflow=off  InputSameDT=off
  Switch1 : Switch  Criteria=u2 > Threshold  SaturateOnIntegerOverflow=off  InputSameDT=off
  rad_pressure : Constant  Value=1358/299792458
  rad_pressure1 : Constant  Value=145/299792458
  F_4 : Outport
  M_4 : Outport  Port=2
  wires:
  MatrixMultiply2/1 -> Sum5/1, Cross Product/2  "F_i"
  MatrixMultiply/1 -> MatrixMultiply2/1
  Sum1/1 -> MatrixMultiply2/2
  s_B/1 -> 1-rho_s/1, Dot Product/2
  1-rho_s/1 -> Sum1/2
  rad_pressure/1 -> Gain/1
  MatrixMultiply1/1 -> Sum1/1
  Constant1/1 -> MatrixMultiply1/1, Dot Product/1
  Gain/1 -> MatrixMultiply/1
  Constant2/1 -> Cross Product/1
  Dot Product/1 -> Switch/1, Switch/2
  Constant/1 -> Switch/3
  Switch/1 -> 2rho_s/1, MatrixMultiply/2
  2rho_s/1 -> Sum/2
  2/3*rho_d/1 -> Sum/1
  Sum/1 -> MatrixMultiply1/2
  Sum3/1 -> MatrixMultiply5/2
  r_N/1 -> 1-rho_s4/1, Dot Product1/2
  1-rho_s4/1 -> Sum3/2
  2rho_s4/1 -> Sum2/2
  Switch1/1 -> 2rho_s4/1, MatrixMultiply3/2
  MatrixMultiply4/1 -> Sum3/1
  Constant5/1 -> Cross Product1/1
  MatrixMultiply3/1 -> MatrixMultiply5/1
  rad_pressure1/1 -> Gain1/1
  Constant3/1 -> Switch1/3
  Constant4/1 -> MatrixMultiply4/1, Dot Product1/1
  MatrixMultiply5/1 -> Sum5/2, Cross Product1/2  "F_i"
  Dot Product1/1 -> Switch1/1, Switch1/2
  Cross Product1/1 -> Sum4/2  "M_i"
  Sum2/1 -> MatrixMultiply4/2
  Gain1/1 -> MatrixMultiply3/1
  2/3*rho_d4/1 -> Sum2/1
  Sum4/1 -> M_4/1
  Cross Product/1 -> Sum4/1  "M_i"
  Sum5/1 -> F_4/1

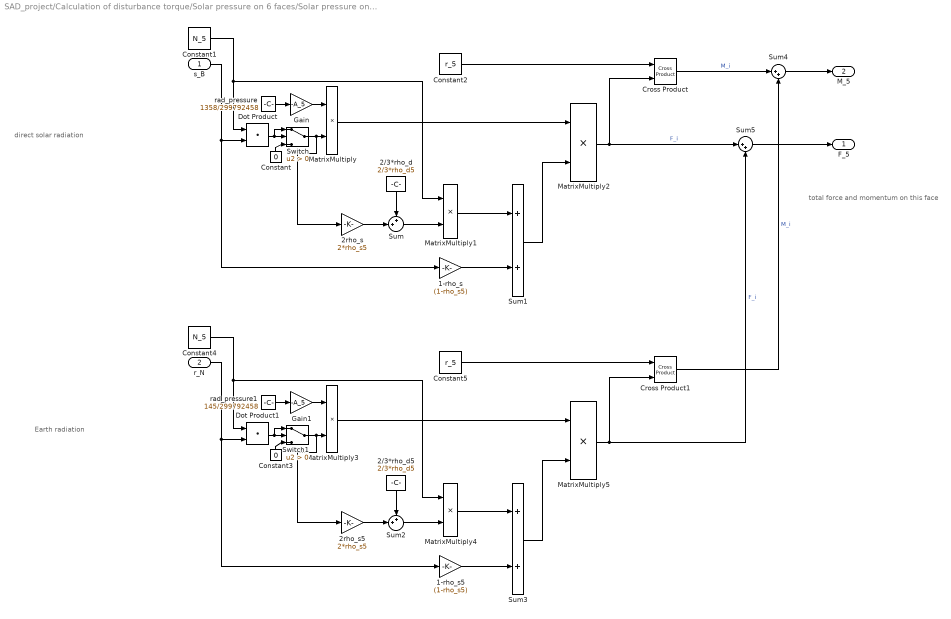
== system SAD_project/Calculation of disturbance torque/Solar pressure on 6 faces/Solar pressure on 6 faces1/solar pressure force and torque 5 ==
  note: total force and
      | momentum on this face
  note: direct solar radiation
  note: Earth radiation
  s_B : Inport
  r_N : Inport  Port=2
  1-rho_s : Gain  Gain=(1-rho_s5)
  1-rho_s5 : Gain  Gain=(1-rho_s5)
  2/3*rho_d : Constant  Value=2/3*rho_d5
  2/3*rho_d5 : Constant  Value=2/3*rho_d5
  2rho_s : Gain  Gain=2*rho_s5
  2rho_s5 : Gain  Gain=2*rho_s5
  Constant : Constant  Value=0
  Constant1 : Constant  Value=N_5
  Constant2 : Constant  Value=r_5
  Constant3 : Constant  Value=0
  Constant4 : Constant  Value=N_5
  Constant5 : Constant  Value=r_5
  Cross Product : matrix_library/Cross Product
  Cross Product1 : matrix_library/Cross Product
  Dot Product : DotProduct  OutDataTypeStr=Inherit: Inherit via internal rule
  Dot Product1 : DotProduct  OutDataTypeStr=Inherit: Inherit via internal rule
  Gain : Gain  Gain=-A_5
  Gain1 : Gain  Gain=-A_5
  MatrixMultiply{,1..5} (6 alike) : Product
  Sum : Sum  Inputs=++|
  Sum1 : Sum
  Sum2 : Sum  Inputs=++|
  Sum3 : Sum
  Sum4 : Sum  Inputs=|++
  Sum5 : Sum  Inputs=|++
  Switch : Switch  Criteria=u2 > Threshold  SaturateOnIntegerOverflow=off  InputSameDT=off
  Switch1 : Switch  Criteria=u2 > Threshold  SaturateOnIntegerOverflow=off  InputSameDT=off
  rad_pressure : Constant  Value=1358/299792458
  rad_pressure1 : Constant  Value=145/299792458
  F_5 : Outport
  M_5 : Outport  Port=2
  wires:
  MatrixMultiply2/1 -> Sum5/1, Cross Product/2  "F_i"
  MatrixMultiply/1 -> MatrixMultiply2/1
  Sum1/1 -> MatrixMultiply2/2
  s_B/1 -> 1-rho_s/1, Dot Product/2
  1-rho_s/1 -> Sum1/2
  rad_pressure/1 -> Gain/1
  MatrixMultiply1/1 -> Sum1/1
  Constant1/1 -> MatrixMultiply1/1, Dot Product/1
  Gain/1 -> MatrixMultiply/1
  Constant2/1 -> Cross Product/1
  Dot Product/1 -> Switch/1, Switch/2
  Constant/1 -> Switch/3
  Switch/1 -> 2rho_s/1, MatrixMultiply/2
  2rho_s/1 -> Sum/2
  2/3*rho_d/1 -> Sum/1
  Sum/1 -> MatrixMultiply1/2
  Sum3/1 -> MatrixMultiply5/2
  r_N/1 -> 1-rho_s5/1, Dot Product1/2
  1-rho_s5/1 -> Sum3/2
  2rho_s5/1 -> Sum2/2
  Switch1/1 -> 2rho_s5/1, MatrixMultiply3/2
  MatrixMultiply4/1 -> Sum3/1
  Constant5/1 -> Cross Product1/1
  MatrixMultiply3/1 -> MatrixMultiply5/1
  rad_pressure1/1 -> Gain1/1
  Constant3/1 -> Switch1/3
  Constant4/1 -> MatrixMultiply4/1, Dot Product1/1
  MatrixMultiply5/1 -> Sum5/2, Cross Product1/2  "F_i"
  Dot Product1/1 -> Switch1/1, Switch1/2
  Cross Product1/1 -> Sum4/2  "M_i"
  Sum2/1 -> MatrixMultiply4/2
  Gain1/1 -> MatrixMultiply3/1
  2/3*rho_d5/1 -> Sum2/1
  Sum4/1 -> M_5/1
  Cross Product/1 -> Sum4/1  "M_i"
  Sum5/1 -> F_5/1

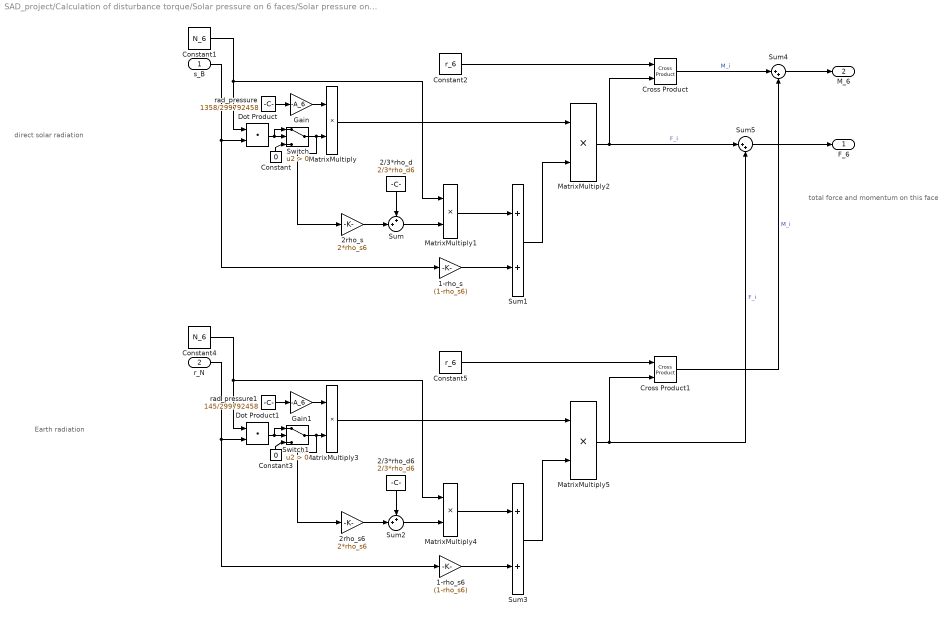
== system SAD_project/Calculation of disturbance torque/Solar pressure on 6 faces/Solar pressure on 6 faces1/solar pressure force and torque 6 ==
  note: total force and
      | momentum on this face
  note: direct solar radiation
  note: Earth radiation
  s_B : Inport
  r_N : Inport  Port=2
  1-rho_s : Gain  Gain=(1-rho_s6)
  1-rho_s6 : Gain  Gain=(1-rho_s6)
  2/3*rho_d : Constant  Value=2/3*rho_d6
  2/3*rho_d6 : Constant  Value=2/3*rho_d6
  2rho_s : Gain  Gain=2*rho_s6
  2rho_s6 : Gain  Gain=2*rho_s6
  Constant : Constant  Value=0
  Constant1 : Constant  Value=N_6
  Constant2 : Constant  Value=r_6
  Constant3 : Constant  Value=0
  Constant4 : Constant  Value=N_6
  Constant5 : Constant  Value=r_6
  Cross Product : matrix_library/Cross Product
  Cross Product1 : matrix_library/Cross Product
  Dot Product : DotProduct  OutDataTypeStr=Inherit: Inherit via internal rule
  Dot Product1 : DotProduct  OutDataTypeStr=Inherit: Inherit via internal rule
  Gain : Gain  Gain=-A_6
  Gain1 : Gain  Gain=-A_6
  MatrixMultiply{,1..5} (6 alike) : Product
  Sum : Sum  Inputs=++|
  Sum1 : Sum
  Sum2 : Sum  Inputs=++|
  Sum3 : Sum
  Sum4 : Sum  Inputs=|++
  Sum5 : Sum  Inputs=|++
  Switch : Switch  Criteria=u2 > Threshold  SaturateOnIntegerOverflow=off  InputSameDT=off
  Switch1 : Switch  Criteria=u2 > Threshold  SaturateOnIntegerOverflow=off  InputSameDT=off
  rad_pressure : Constant  Value=1358/299792458
  rad_pressure1 : Constant  Value=145/299792458
  F_6 : Outport
  M_6 : Outport  Port=2
  wires:
  MatrixMultiply2/1 -> Sum5/1, Cross Product/2  "F_i"
  MatrixMultiply/1 -> MatrixMultiply2/1
  Sum1/1 -> MatrixMultiply2/2
  s_B/1 -> 1-rho_s/1, Dot Product/2
  1-rho_s/1 -> Sum1/2
  rad_pressure/1 -> Gain/1
  MatrixMultiply1/1 -> Sum1/1
  Constant1/1 -> MatrixMultiply1/1, Dot Product/1
  Gain/1 -> MatrixMultiply/1
  Constant2/1 -> Cross Product/1
  Dot Product/1 -> Switch/1, Switch/2
  Constant/1 -> Switch/3
  Switch/1 -> 2rho_s/1, MatrixMultiply/2
  2rho_s/1 -> Sum/2
  2/3*rho_d/1 -> Sum/1
  Sum/1 -> MatrixMultiply1/2
  Sum3/1 -> MatrixMultiply5/2
  r_N/1 -> 1-rho_s6/1, Dot Product1/2
  1-rho_s6/1 -> Sum3/2
  2rho_s6/1 -> Sum2/2
  Switch1/1 -> 2rho_s6/1, MatrixMultiply3/2
  MatrixMultiply4/1 -> Sum3/1
  Constant5/1 -> Cross Product1/1
  MatrixMultiply3/1 -> MatrixMultiply5/1
  rad_pressure1/1 -> Gain1/1
  Constant3/1 -> Switch1/3
  Constant4/1 -> MatrixMultiply4/1, Dot Product1/1
  MatrixMultiply5/1 -> Sum5/2, Cross Product1/2  "F_i"
  Dot Product1/1 -> Switch1/1, Switch1/2
  Cross Product1/1 -> Sum4/2  "M_i"
  Sum2/1 -> MatrixMultiply4/2
  Gain1/1 -> MatrixMultiply3/1
  2/3*rho_d6/1 -> Sum2/1
  Sum4/1 -> M_6/1
  Cross Product/1 -> Sum4/1  "M_i"
  Sum5/1 -> F_6/1

== system SAD_project/Dynamics e Kinematics/Attitude error GG/calculating A_B//L/Subsystem ==
  note: A_L/N=A3(om+th)A1(i)A3(OM)
  Theta : Inport
  Constant : Constant  Value=[1,0,0;0 cos(i) sin(i); 0 -sin(i) cos(i)]
  Constant1 : Constant
  Constant2 : Constant  Value=0
  Constant3 : Constant  Value=om
  Constant4 : Constant  Value=[cos(OM),sin(OM),0;-sin(OM),cos(OM),0;0,0,1]
  Cos : Trigonometry  Operator=cos
  Gain : Gain  Gain=-1
  Matrix Concatenate : Concatenate  NumInputs=3  Mode=Multidimensional array  ConcatenateDimension=2
  Matrix Multiply : Product  Inputs=3  Multiplication=Matrix(*)
  Sin : Trigonometry
  Sum : Sum  Inputs=|++
  Vector Concatenate : Concatenate  NumInputs=3
  Vector Concatenate1 : Concatenate  NumInputs=3
  Vector Concatenate2 : Concatenate  NumInputs=3
  " A_L/N" : Outport
  wires:
  Vector Concatenate/1 -> Matrix Concatenate/1
  Vector Concatenate2/1 -> Matrix Concatenate/3
  Matrix Concatenate/1 -> Matrix Multiply/1
  Matrix Multiply/1 -> " A_L/N"/1
  Sin/1 -> Gain/1, Vector Concatenate1/1
  Gain/1 -> Vector Concatenate/2
  Vector Concatenate1/1 -> Matrix Concatenate/2
  Cos/1 -> Vector Concatenate/1, Vector Concatenate1/2
  Constant1/1 -> Vector Concatenate2/3
  Constant/1 -> Matrix Multiply/2
  Constant2/1 -> Vector Concatenate/3, Vector Concatenate1/3, Vector Concatenate2/1, Vector Concatenate2/2
  Theta/1 -> Sum/1
  Sum/1 -> Cos/1, Sin/1
  Constant3/1 -> Sum/2
  Constant4/1 -> Matrix Multiply/3

== system SAD_project/Subsystem/Switch Case Action Adavanced Magnetic model/Advanced magnetic field model/Rotation matrix for earth spin ==
  Clock1 : Clock
  Constant22 : Constant  Value=n_e
  Product3 : Product
  Rotation matrix 3 : Subsystem
  eci_to_ecef : Outport
  wires:
  Rotation matrix 3/1(theta_mat) -> eci_to_ecef/1
  Product3/1 -> Rotation matrix 3/1(In1)
  Constant22/1 -> Product3/1
  Clock1/1 -> Product3/2

== system SAD_project/Subsystem/Switch Case Action Adavanced Magnetic model/Advanced magnetic field model/cart to sph coord ==
  r_xyz : Inport
  Atan1 : Trigonometry  Operator=atan2
  Atan2 : Trigonometry  Operator=atan2
  Demux : Demux  Outputs=3
  Dot Product : DotProduct  OutDataTypeStr=Inherit: Inherit via internal rule
  Sqrt : Sqrt
  Square : Math  Operator=square
  Square Root : Sqrt
  Square1 : Math  Operator=square
  Sum : Sum  Inputs=|++
  r : Outport
  lat : Outport  Port=2
  long : Outport  Port=3
  wires:
  r_xyz/1 -> Dot Product/2, Dot Product/1, Demux/1
  Demux/2 -> Square/1, Atan2/1
  Demux/1 -> Atan2/2, Square1/1
  Atan2/1 -> long/1
  Demux/3 -> Atan1/1
  Square1/1 -> Sum/1
  Square/1 -> Sum/2
  Sum/1 -> Square Root/1
  Square Root/1 -> Atan1/2
  Atan1/1 -> lat/1
  Dot Product/1 -> Sqrt/1
  Sqrt/1 -> r/1

== system SAD_project/Subsystem/Switch Case Action Dipole model/Dipol Model of Magnetic Field/Calculation of b_n ==
  H0 vector : Inport
  EarthSat_n : Inport  Port=2
  Constant : Constant  Value=3
  Divide : Product  Inputs=*/
  Dot Product : DotProduct  OutDataTypeStr=Inherit: Inherit via internal rule
  Gain : Gain  Gain=3
  Gain1 : Gain  Gain=R_E^3
  Norm of Vector : Subsystem  AncestorBlock=LibrarySAD5/Normalize Vector1
  Norm of Vector H : Subsystem  AncestorBlock=LibrarySAD5/Normalize Vector1
  Normalize Vector : Subsystem
  Power : Math  Operator=pow
  Product : Product
  Product1 : Product
  Subtract : Sum  Inputs=+-
  m_versor : Subsystem
  b_N : Outport
  wires:
  Norm of Vector/1(Norm) -> Power/1
  Product/1 -> Subtract/1
  Divide/1 -> Gain1/1
  EarthSat_n/1 -> Norm of Vector/1(Vector), Normalize Vector/1(Vector)
  Normalize Vector/1(Versor) -> Product/1, Dot Product/1
  Gain1/1 -> Product1/1
  m_versor/1(m_versor) -> Dot Product/2, Subtract/2
  Gain/1 -> Product/2
  Product1/1 -> b_N/1
  Constant/1 -> Power/2
  Dot Product/1 -> Gain/1
  Subtract/1 -> Product1/2
  Norm of Vector H/1(Norm) -> Divide/1
  Power/1 -> Divide/2
  H0 vector/1 -> Norm of Vector H/1(Vector)

== system SAD_project/TRIAD: Attitude determination algebric Method with 2 sensor/Subsystem/Normalize Vector3/Normalize Vector ==
  Vector : Inport
  Dot Product : DotProduct  OutDataTypeStr=Inherit: Inherit via internal rule
  Sqrt : Sqrt
  Norm : Outport
  wires:
  Sqrt/1 -> Norm/1
  Vector/1 -> Dot Product/1, Dot Product/2
  Dot Product/1 -> Sqrt/1

== system SAD_project/TRIAD: Attitude determination algebric Method with 2 sensor/Subsystem1/Normalize Vector3/Normalize Vector ==
  Vector : Inport
  Dot Product : DotProduct  OutDataTypeStr=Inherit: Inherit via internal rule
  Sqrt : Sqrt
  Norm : Outport
  wires:
  Sqrt/1 -> Norm/1
  Vector/1 -> Dot Product/1, Dot Product/2
  Dot Product/1 -> Sqrt/1

== system SAD_project/Subsystem/Switch Case Action Adavanced Magnetic model/Advanced magnetic field model/Rotation matrix for earth spin/Rotation matrix 3 ==
  In1 : Inport
  Constant1 : Constant  Value=[0 0 0; 0 0 0; 0 0 1]
  Cos2 : Trigonometry  Operator=cos
  Gain : Gain  Gain=[1 0 0; 0 1 0; 0 0 0]
  Gain1 : Gain  Gain=[0 1 0; -1 0 0; 0 0 0]
  Sin2 : Trigonometry
  Sum : Sum  Inputs=+++
  theta_mat : Outport
  wires:
  Cos2/1 -> Gain/1
  Gain/1 -> Sum/1
  In1/1 -> Sin2/1, Cos2/1
  Sin2/1 -> Gain1/1
  Sum/1 -> theta_mat/1
  Gain1/1 -> Sum/2
  Constant1/1 -> Sum/3

== system SAD_project/Subsystem/Switch Case Action Dipole model/Dipol Model of Magnetic Field/Calculation of b_n/Norm of Vector ==
  Vector : Inport
  Dot Product : DotProduct  OutDataTypeStr=Inherit: Inherit via internal rule
  Sqrt : Sqrt
  Norm : Outport
  wires:
  Sqrt/1 -> Norm/1
  Vector/1 -> Dot Product/1, Dot Product/2
  Dot Product/1 -> Sqrt/1

== system SAD_project/Subsystem/Switch Case Action Dipole model/Dipol Model of Magnetic Field/Calculation of b_n/Norm of Vector H ==
  Vector : Inport
  Dot Product : DotProduct  OutDataTypeStr=Inherit: Inherit via internal rule
  Sqrt : Sqrt
  Norm : Outport
  wires:
  Sqrt/1 -> Norm/1
  Vector/1 -> Dot Product/1, Dot Product/2
  Dot Product/1 -> Sqrt/1

== system SAD_project/Subsystem/Switch Case Action Dipole model/Dipol Model of Magnetic Field/Calculation of b_n/Normalize Vector ==
  Vector : Inport
  Divide : Product  Inputs=*/
  Normalize Vector1 : Subsystem  AncestorBlock=LibrarySAD5/Normalize Vector1
  Versor : Outport
  wires:
  Vector/1 -> Normalize Vector1/1(Vector), Divide/1
  Divide/1 -> Versor/1
  Normalize Vector1/1(Norm) -> Divide/2

== system SAD_project/Subsystem/Switch Case Action Dipole model/Dipol Model of Magnetic Field/Calculation of b_n/m_versor ==
  Clock : Clock
  Constant : Constant  Value=cos(deg2rad(11.5))
  Cos : Trigonometry  Operator=cos
  Gain : Gain  Gain=deg2rad(w_E)
  Gain1 : Gain  Gain=sin(deg2rad(11.5))
  Gain2 : Gain  Gain=sin(deg2rad(11.5))
  Sin : Trigonometry
  Vector Concatenate : Concatenate  NumInputs=3
  m_versor : Outport
  wires:
  Clock/1 -> Gain/1
  Gain/1 -> Sin/1, Cos/1
  Gain2/1 -> Vector Concatenate/2
  Vector Concatenate/1 -> m_versor/1
  Cos/1 -> Gain1/1
  Constant/1 -> Vector Concatenate/3
  Sin/1 -> Gain2/1
  Gain1/1 -> Vector Concatenate/1

== system SAD_project/Subsystem/Switch Case Action Dipole model/Dipol Model of Magnetic Field/Calculation of b_n/Normalize Vector/Normalize Vector1 ==
  Vector : Inport
  Dot Product : DotProduct  OutDataTypeStr=Inherit: Inherit via internal rule
  Sqrt : Sqrt
  Norm : Outport
  wires:
  Sqrt/1 -> Norm/1
  Vector/1 -> Dot Product/1, Dot Product/2
  Dot Product/1 -> Sqrt/1

== matlab function SAD_project/Subsystem/Switch Case Action Adavanced Magnetic model/Advanced magnetic field model/MATLAB Function ==
  data: r input; B_n output; theta input; phi input; LST input; mjd2000 input; A1 input; A2 input; N input
function B_n = magnetic_field_model(r,theta,phi, LST, mjd2000, A1, A2, N)

%   mjd2000[1]  Date in MJD 2000. MJD2000 is defined as the number of days
%               since 01-01-2000, 12:00 noon.
days = mjd2000 - 7305;      % 7305 is the Julian time from 2000 to 2020

% Inputs
% r         Geocentric radius
% theta     Latitude measured in degrees positive from equator  
% phi       Longitude measured in degrees positive east from Greenwich
% days      Decimal days since January 1, 2020
% N         Order of expansion of the magnetic field model
%
% Outputs - magnetic field strength in local tangential coordinates
% Br    B in radial direction
% Bt    B in theta direction
% Bp    B in phi direction
[Br,Bt,Bp] = magnet(r,theta,phi,days, N, A1, A2);

% Inputs
% Br    B in radial direction
% Bt    B in theta direction
% Bp    B in phi direction
% LST   Local sidereal time of location (in degrees)(right ascension)
% lat   Latitude measured positive north from equator (in degrees), it is
%       the same as the local declination
%
% Outputs
% Bx    B in x-direction  | Magnetic field strength (B)
% By    B in y-direction  | in geocentric inertial coordinates
% Bz    B in z-direction  |
[Bx,By,Bz] = msph2inert(Br,Bt,Bp,LST, theta);

B_n = [Bx,By,Bz]';
